simulink model "LCK_0112"  (R2018b)
settings: Solver=FixedStepDiscrete  StartTime=0.0  StopTime=inf  FixedStep=0.01  RelTol=1e-3
PostLoadFcn:
  | if any(exist('dsrtsu_mdlpostloadfcn', 'file') ~= 0), dsrtsu_mdlpostloadfcn('Execute', bdroot); end
values from neighbouring files (symbols this model uses):
  C_DEG2RAD = 0.0175    [LCK_Macro.sldd]
  C_KPH2MPS = 0.2778    [LCK_Macro.sldd]
  C_NEARZERO = 0.0001    [LCK_Macro.sldd]
  C_ONE = 1.0    [LCK_Macro.sldd]
  C_RAD2DEG = 57.2958    [LCK_Macro.sldd]
  C_ZERO = 0.0    [LCK_Macro.sldd]
  k_accel_pedal_pos_per_speed_x : value not decoded    [LCK_LogicPara.sldd]
  k_accel_pedal_pos_per_speed_z : value not decoded    [LCK_LogicPara.sldd]
  k_brake_suprress_hold = 1000.0    [LCK_LogicPara.sldd]
  k_driver_appl_torque_filt = 50.0    [LCK_LogicPara.sldd]
  k_driver_suppression_hold_time = 3000.0    [LCK_LogicPara.sldd]
  k_hands_on_wheel_hold_msec = 500.0    [LCK_LogicPara.sldd]
  k_hands_on_wheel_torque_hi = 0.2    [LCK_LogicPara.sldd]
  k_hands_on_wheel_torque_lo = 0.15    [LCK_LogicPara.sldd]
  k_handsoff_delay_cycles = 50.0    [LCK_LogicPara.sldd]
  k_handsoff_torq_Lo_CR = 0.3    [LCK_LogicPara.sldd]
  k_handson_delay_cycles = 5.0    [LCK_LogicPara.sldd]
  k_HighAccel_suppress_hold = 3000.0    [LCK_LogicPara.sldd]
  k_HLR_suprress_hold = 3000.0    [LCK_LogicPara.sldd]
  k_hs_StrAng_CR_threshold_z : value not decoded    [LCK_LogicPara.sldd]
  k_LC_Exit_Switch = 0.0    [LCK_LogicPara.sldd]
  k_LCG_Configured = 1.0    [LCK_LogicPara.sldd]
  k_LCK_A0_Rdy2Act_UseConst = 0.0    [LCK_LogicPara.sldd]
  k_LCK_A0Fac_ActSta : value not decoded    [LCK_CtrlPara.sldd]
  k_LCK_A0Fac_DrvStm : value not decoded    [LCK_CtrlPara.sldd]
  k_LCK_A0Shift_LftCurv : value not decoded    [LCK_CtrlPara.sldd]
  k_LCK_A0Shift_RgtCurv : value not decoded    [LCK_CtrlPara.sldd]
  k_LCK_A0Shift_StraLan = 0.0    [LCK_CtrlPara.sldd]
  k_LCK_A0ShiftFac_Dy_LftCurv : value not decoded    [LCK_CtrlPara.sldd]
  k_LCK_A0ShiftFac_Dy_RgtCurv : value not decoded    [LCK_CtrlPara.sldd]
  k_LCK_A0ShiftFac_Vspd : value not decoded    [LCK_CtrlPara.sldd]
  k_LCK_accel_inhibit_thold = 35.0    [LCK_LogicPara.sldd]
  k_LCK_Active2Ready_Mask = 255.0    [LCK_LogicPara.sldd]
  k_LCK_CvatRateBks : value not decoded    [LCK_CtrlPara.sldd]
  k_LCK_CvatrBks : value not decoded    [LCK_CtrlPara.sldd]
  k_LCK_DFac_Dy : value not decoded    [LCK_CtrlPara.sldd]
  k_LCK_DFac_Dy_Curv : value not decoded    [LCK_CtrlPara.sldd]
  k_LCK_DFac_HaCurCen : value not decoded    [LCK_CtrlPara.sldd]
  k_LCK_DFac_HaCurSid : value not decoded    [LCK_CtrlPara.sldd]
  k_LCK_DFac_HadCurCen : value not decoded    [LCK_CtrlPara.sldd]
  k_LCK_DFac_HadCurSid : value not decoded    [LCK_CtrlPara.sldd]
  k_LCK_DFac_HadStrCen : value not decoded    [LCK_CtrlPara.sldd]
  k_LCK_DFac_HadStrSid : value not decoded    [LCK_CtrlPara.sldd]
  k_LCK_DFac_HaStrCen : value not decoded    [LCK_CtrlPara.sldd]
  k_LCK_DFac_HaStrSid : value not decoded    [LCK_CtrlPara.sldd]
  k_LCK_DFac_Rad : value not decoded    [LCK_CtrlPara.sldd]
  k_LCK_DFac_SA_CurCen : value not decoded    [LCK_CtrlPara.sldd]
  k_LCK_DFac_SA_CurSid : value not decoded    [LCK_CtrlPara.sldd]
  k_LCK_DFac_SA_StrCen : value not decoded    [LCK_CtrlPara.sldd]
  k_LCK_DFac_SA_StrSid : value not decoded    [LCK_CtrlPara.sldd]
  k_LCK_DFac_SS_CurCen : value not decoded    [LCK_CtrlPara.sldd]
  k_LCK_DFac_SS_CurSid : value not decoded    [LCK_CtrlPara.sldd]
  k_LCK_DFac_SS_StrCen : value not decoded    [LCK_CtrlPara.sldd]
  k_LCK_DFac_SS_StrSid : value not decoded    [LCK_CtrlPara.sldd]
  k_LCK_DFac_Vspd : value not decoded    [LCK_CtrlPara.sldd]
  k_LCK_DlyTm_DrvStim = 0.2    [LCK_CtrlPara.sldd]
  k_LCK_DTermMax = 2.0    [LCK_CtrlPara.sldd]
  k_LCK_DyBks_Curv : value not decoded    [LCK_CtrlPara.sldd]
  k_LCK_Enable_POOnly = 1.0    [LCK_LogicPara.sldd]
  k_LCK_Entry_DistBuffer = 0.1    [LCK_LogicPara.sldd]
  k_LCK_Fac_Vspd2RngThr_FalRec = 0.23    [LCK_CtrlPara.sldd]
  k_LCK_Ffw_CvatSwh = 0.0    [LCK_CtrlPara.sldd]
  k_LCK_Ffw_DyBks : value not decoded    [LCK_CtrlPara.sldd]
  k_LCK_Ffw_TimCon_CmdFlt = 0.0    [LCK_CtrlPara.sldd]
  k_LCK_FfwDeltaFac_Rad_Lft : value not decoded    [LCK_CtrlPara.sldd]
  k_LCK_FfwDeltaFac_Rad_Rgt : value not decoded    [LCK_CtrlPara.sldd]
  k_LCK_FfwDeltaFac_Vspd : value not decoded    [LCK_CtrlPara.sldd]
  k_LCK_FfwFac_CvatRate_Lft : value not decoded    [LCK_CtrlPara.sldd]
  k_LCK_FfwFac_CvatRate_Rgt : value not decoded    [LCK_CtrlPara.sldd]
  k_LCK_FfwFac_Dy : value not decoded    [LCK_CtrlPara.sldd]
  k_LCK_FfwFac_Rad_Lft : value not decoded    [LCK_CtrlPara.sldd]
  k_LCK_FfwFac_Rad_Rgt : value not decoded    [LCK_CtrlPara.sldd]
  k_LCK_FfwFac_Vspd : value not decoded    [LCK_CtrlPara.sldd]
  k_LCK_FfwTorq_Cvat : value not decoded    [LCK_CtrlPara.sldd]
  k_LCK_HAFac_ActSta : value not decoded    [LCK_CtrlPara.sldd]
  k_LCK_HAFac_DrvStm : value not decoded    [LCK_CtrlPara.sldd]
  k_LCK_HaloTime = 2000.0    [LCK_LogicPara.sldd]
  k_LCK_HaloTime_Switch = 0.0    [LCK_LogicPara.sldd]
  k_LCK_HARFac_ActSta : value not decoded    [LCK_CtrlPara.sldd]
  k_LCK_HARFac_DrvStm : value not decoded    [LCK_CtrlPara.sldd]
  k_LCK_Hed_DyBks : value not decoded    [LCK_CtrlPara.sldd]
  k_LCK_HedAngDiffX : value not decoded    [LCK_CtrlPara.sldd]
  k_LCK_HedAngRateDiffX : value not decoded    [LCK_CtrlPara.sldd]
  k_LCK_HndsOnWhel_DlyTm_Idl2Rdy = 0.0    [LCK_LogicPara.sldd]
  k_LCK_host_veh_width = 1.86    [LCK_LogicPara.sldd]
  k_LCK_Idle2Ready_Mask = 239.0    [LCK_LogicPara.sldd]
  k_LCK_Junc_SusTime = 1.0    [LCK_LogicPara.sldd]
  k_LCK_KpKdDecSlopeLmt = 10.0    [LCK_CtrlPara.sldd]
  k_LCK_KpKdIncSlopeLmt = 5.0    [LCK_CtrlPara.sldd]
  k_LCK_Lat_Ctrl_DFac_Lft = 1.0    [LCK_CtrlPara.sldd]
  k_LCK_Lat_Ctrl_DFac_Rgt = 1.05    [LCK_CtrlPara.sldd]
  k_LCK_Lat_Ctrl_Kd = 0.8    [LCK_CtrlPara.sldd]
  k_LCK_Lat_Ctrl_Ki = 0.5    [LCK_CtrlPara.sldd]
  k_LCK_Lat_Ctrl_Kp = 0.7    [LCK_CtrlPara.sldd]
  k_LCK_Lat_Ctrl_Kp_NearGain = 0.7    [LCK_CtrlPara.sldd]
  k_LCK_Lat_Ctrl_PFac_Lft = 1.0    [LCK_CtrlPara.sldd]
  k_LCK_Lat_Ctrl_PFac_Rgt = 1.05    [LCK_CtrlPara.sldd]
  k_LCK_Lat_Ctrl_TimCon_CmdFlt = 5.0    [LCK_CtrlPara.sldd]
  k_LCK_Lat_DFac_Rad : value not decoded    [LCK_CtrlPara.sldd]
  k_LCK_Lat_DFac_SS_Cur : value not decoded    [LCK_CtrlPara.sldd]
  k_LCK_Lat_DFac_SS_Str : value not decoded    [LCK_CtrlPara.sldd]
  k_LCK_Lat_DFac_Vspd : value not decoded    [LCK_CtrlPara.sldd]
  k_LCK_Lat_DyBks : value not decoded    [LCK_CtrlPara.sldd]
  k_LCK_Lat_IFac_Rad : value not decoded    [LCK_CtrlPara.sldd]
  k_LCK_Lat_IFac_Vspd : value not decoded    [LCK_CtrlPara.sldd]
  k_LCK_Lat_ILmtFac_Dy_CurvLan : value not decoded    [LCK_CtrlPara.sldd]
  k_LCK_Lat_ILmtFac_Dy_StraLan : value not decoded    [LCK_CtrlPara.sldd]
  k_LCK_Lat_ILmtFac_Rad : value not decoded    [LCK_CtrlPara.sldd]
  k_LCK_Lat_ILmtFac_Rad_NearGain = 1.0    [LCK_CtrlPara.sldd]
  k_LCK_Lat_ILmtFac_Vspd_CurvLan : value not decoded    [LCK_CtrlPara.sldd]
  k_LCK_Lat_ILmtFac_Vspd_StraLan : value not decoded    [LCK_CtrlPara.sldd]
  k_LCK_Lat_ITermLmt_Dy = 1.0    [LCK_CtrlPara.sldd]
  k_LCK_Lat_KpKdDecSlopeLmt = 10.0    [LCK_CtrlPara.sldd]
  k_LCK_Lat_KpKdIncSlopeLmt = 10.0    [LCK_CtrlPara.sldd]
  k_LCK_Lat_PFac_Dy_InnLftCur : value not decoded    [LCK_CtrlPara.sldd]
  k_LCK_Lat_PFac_Dy_InnRgtCur : value not decoded    [LCK_CtrlPara.sldd]
  k_LCK_Lat_PFac_Dy_OutLftCur : value not decoded    [LCK_CtrlPara.sldd]
  k_LCK_Lat_PFac_Dy_OutRgtCur : value not decoded    [LCK_CtrlPara.sldd]
  k_LCK_Lat_PFac_Dy_Str : value not decoded    [LCK_CtrlPara.sldd]
  k_LCK_Lat_PFac_Rad : value not decoded    [LCK_CtrlPara.sldd]
  ... (+153 more)
undefined symbols (not defined in the file or in its folder): k_LCK_CurvBks, K_LCK_SPA0A1A2_LMRngCmp_y
libraries: LateralControl_fcns_lib x58, simulink x24
(part 35 of 45)

== system LCK_0112/Lateral_Control_Module/LCK_State_Ctrl/LCK_Mode_Transition/Yaw_Rate_Judgement ==
  yaw_deg_iso_filt : Inport
  SP_A2 : Inport  Port=2
  Abs17 : Abs  Tag={'output',{'type','Float32'},'date',737463.83860062505}  Description=_GWMH9P4.LCK.000_47_
  Abs18 : Abs  Tag={'output',{'type','Float32'},'date',737463.83780197916}  Description=_GWMH9P4.LCK.000_48_  OutDataTypeStr=single
  C_NEARZERO : Constant  Tag={'output',{'name','$P','class','EXTERN_CONST','type','Float32'},'date',737463.83784295141}  Description=_GWMH9P4.LCK.000_49_  Value=C_NEARZERO
  Constant54 : Constant  Tag={'output',{'type','Int32'},'date',737462.50906520837}  Description=_GWMH9P4.LCK.000_52_
  Data Type Conversion86 : DataTypeConversion  Description=_GWMH9P4.LCK.000_70_
  Delay_Trig : LateralControl_fcns_lib/Delay_Trig  SystemSampleTime=-1
  Divide : Product  Tag={'output',{'type','Float32'},'exceptionhandling',0,'date',737477.59124685184}  Description=_GWMH9P4.LCK.000_71_  Inputs=*/
  First_Order_Lag_Filter2 : Subsystem  TreatAsAtomicUnit=on
  Gain17 : Gain  Tag={'output',{'type','Float32'},'gain',{'type','Int32'},'date',737463.83831937495}  Description=_GWMH9P4.LCK.000_85_  Gain=2
  ML_TIME_MSEC : Constant  Tag={'output',{'name','$P','class','EXTERN_MACRO','type','ESR_Typedefs/unsigned8_T'},'date',737462.69417359959}  Description=_GWMH9P4.LCK.000_129_  Value=ML_TIME_MSEC
  MinMax : MinMax  Tag={'output',{'type','Float32'},'date',737463.83775070601}  Description=_GWMH9P4.LCK.000_130_  Function=max  Inputs=2
  Relational Operator201 : RelationalOperator  Tag={'date',737462.50909680559}  Description=_GWMH9P4.LCK.000_136_  Operator=>  OutDataTypeStr=boolean  RndMeth=Nearest
  k_LCK_ROC_filt_tau : Constant  Tag={'output',{'name','$P','class','EXTERN_CAL','type','UInt16'},'date',737531.64282156248}  Description=_GACA26P4.LCK.000_61_  Value=k_LCK_ROC_filt_tau
  k_LCK_YawRateThr_Act2Rdy : Lookup_n-D  Tag={'input',{'name','$P','class','EXTERN_CAL','type','Float32'},'output',{'type','Float32'},'table',{'name','$P','class','EXTERN_CAL','type','Float32'},'date',737463.83819582174}  Description=_GWMH9P4.LCK.000_176_  NumberOfTableDimensions=1  BreakpointsForDimension1=k_LCK_YawRateThr_Act2Rdy_ROC_x  IndexSearchMethod=Linear search  Table=k_LCK_YawRateThr_Act2Rdy_z  ExtrapMethod=Clip  InputSameDT=on
  k_LCK_YawRateThr_DlyTm_Act2Rdy : Constant  Tag={'output',{'name','$P','class','EXTERN_CAL','type','Float32'},'date',737469.66737693292}  Description=_GWMH9P4.LCK.000_177_  Value=k_LCK_YawRateThr_DlyTm_Act2Rdy
  YawRate_Over_Threshold : Outport
  wires:
  First_Order_Lag_Filter2/1(filtered_output) -> k_LCK_YawRateThr_Act2Rdy/1
  Delay_Trig/1 -> YawRate_Over_Threshold/1
  Abs18/1 -> MinMax/1
  Divide/1 -> First_Order_Lag_Filter2/1(unfiltered_input)
  k_LCK_ROC_filt_tau/1 -> First_Order_Lag_Filter2/2(filt_tau_msec)
  Gain17/1 -> Abs18/1
  ML_TIME_MSEC/1 -> First_Order_Lag_Filter2/3(filt_loop_time_msec)
  C_NEARZERO/1 -> MinMax/2
  Constant54/1 -> Divide/1
  k_LCK_YawRateThr_Act2Rdy/1 -> Relational Operator201/2
  k_LCK_YawRateThr_DlyTm_Act2Rdy/1 -> Delay_Trig/2
  Data Type Conversion86/1 -> Delay_Trig/1
  Abs17/1 -> Relational Operator201/1
  MinMax/1 -> Divide/2
  Relational Operator201/1 -> Data Type Conversion86/1
  SP_A2/1 -> Gain17/1
  yaw_deg_iso_filt/1 -> Abs17/1

== system LCK_0112/RTI Data/RTI Data Store/RTI Data Store/RTI Data Store ==
  RTI Data Store : Subsystem  mask(RTI_DATA_STORE){}
      mask help:
      | RTI Data Store Block. This block is used by RTI to store internal model dependent data. Deleting this block will result in data loss.
      |
      | NEVER DELETE, COPY, OR MODIFY THIS BLOCK!
      mask Help:
      | RTI Data Store Block. This block is used by RTI to store internal model dependent data. Deleting this block will result in data loss.
      | 
      | NEVER DELETE, COPY, OR MODIFY THIS BLOCK!
      mask Display: text(0.5, 0.5, ' ', 'HorizontalAlignment', 'center');

== system LCK_0112/Lateral_Control_Module/Adas_Lateral_Control_LCK_Core/Module 3/Sig_Wekng_0/Trigger Hold Counter ==
  Trigger : Inport  Description=_GACA26P4.LCK.000_235_  OutDataTypeStr=boolean
  hold_time : Inport  Description=_GACA26P4.LCK.000_236_  Port=2  OutDataTypeStr=single
  Trigger Hold : Stateflow chart  TreatAsAtomicUnit=on
  Out : Outport  Description=_GACA26P4.LCK.000_241_  OutDataTypeStr=boolean
  Counter : Outport  Description=_GACA26P4.LCK.000_242_  Port=2  OutDataTypeStr=single
  wires:
  Trigger Hold/2(count) -> Counter/1
  Trigger/1 -> Trigger Hold/1(Trigger)
  hold_time/1 -> Trigger Hold/2(hold_time)
  Trigger Hold/1(Out) -> Out/1

== system LCK_0112/Lateral_Control_Module/Adas_Lateral_Control_LCK_Core/Module 8/Module 0/D Gain ==
  LatCtrl_DFac_Asym : Inport
  LatCtrl_DFac_Vspd : Inport  Port=2
  LatCtrl_DFac_Radius : Inport  Port=3
  LatCtrl_DFac_StrSpd : Inport  Port=4
  Product : Product  Inputs=5
  k_LCK_Lat_Ctrl_Kd : Constant  Value=k_LCK_Lat_Ctrl_Kd
  D_Gain : Outport
  wires:
  Product/1 -> D_Gain/1
  LatCtrl_DFac_Asym/1 -> Product/2
  k_LCK_Lat_Ctrl_Kd/1 -> Product/1
  LatCtrl_DFac_Vspd/1 -> Product/3
  LatCtrl_DFac_Radius/1 -> Product/4
  LatCtrl_DFac_StrSpd/1 -> Product/5

== system LCK_0112/Lateral_Control_Module/Adas_Lateral_Control_LCK_Core/Module 8/Module 0/Definition  Fac 1  ==
  Dy_1 : Inport
  Dy_0 : Inport  Port=2
  Lat_Rate : Inport  Port=3
  Relay : Relay  OnSwitchValue=0.02  OffSwitchValue=-0.02
  Relay1 : Relay  OnSwitchValue=0.02  OffSwitchValue=-0.02
  Relay2 : Relay  OnSwitchValue=0.02  OffSwitchValue=-0.02
  Switch1 : Switch  Criteria=u2 > Threshold
  Switch15 : Switch  Criteria=u2 > Threshold
  Switch25 : Switch  Criteria=u2 > Threshold
  k_LCK_Lat_Ctrl_DFac_Lft : Constant  Value=k_LCK_Lat_Ctrl_DFac_Lft
  k_LCK_Lat_Ctrl_DFac_Rgt : Constant  Value=k_LCK_Lat_Ctrl_DFac_Rgt
  k_LCK_Lat_Ctrl_PFac_Lft : Constant  Value=k_LCK_Lat_Ctrl_PFac_Lft
  k_LCK_Lat_Ctrl_PFac_Rgt : Constant  Value=k_LCK_Lat_Ctrl_PFac_Rgt
  LatCtrl_P0Fac_Asym : Outport
  LatCtrl_P1Fac_Asym : Outport  Port=2
  LatCtrl_DFac_Asym : Outport  Port=3
  wires:
  Lat_Rate/1 -> Relay2/1
  Relay/1 -> Switch25/2
  Switch1/1 -> LatCtrl_DFac_Asym/1
  Relay2/1 -> Switch1/2
  Relay1/1 -> Switch15/2
  k_LCK_Lat_Ctrl_PFac_Rgt/1 -> Switch15/1, Switch25/1
  k_LCK_Lat_Ctrl_DFac_Rgt/1 -> Switch1/1
  k_LCK_Lat_Ctrl_PFac_Lft/1 -> Switch25/3, Switch15/3
  k_LCK_Lat_Ctrl_DFac_Lft/1 -> Switch1/3
  Switch15/1 -> LatCtrl_P1Fac_Asym/1
  Switch25/1 -> LatCtrl_P0Fac_Asym/1
  Dy_1/1 -> Relay1/1
  Dy_0/1 -> Relay/1
